simulink model "PID_quadricottero_v3"  (R2023b)
settings: Solver=VariableStepAuto  StartTime=0.0  StopTime=30  RelTol=1e-3
values from neighbouring files (symbols this model uses):
  b = 1.3e-5    (= 1.3e-05)    [data_quadricottero.m]
  d = 1.39e-6    (= 1.39e-06)    [data_quadricottero.m]
  g = 9.8    [data_quadricottero.m]
  Ix = 0.4    [data_quadricottero.m]
  Iy = 0.4    [data_quadricottero.m]
  Iz = 0.7    [data_quadricottero.m]
  l = 0.2    [data_quadricottero.m]
  m = 10    [data_quadricottero.m]
  p0 = 0    [data_quadricottero.m]
  phi0 = 0    [data_quadricottero.m]
  psi0 = 0    [data_quadricottero.m]
  q0 = 0    [data_quadricottero.m]
  r0 = 0    [data_quadricottero.m]
  Tc_Mx = 0.052    [data_quadricottero.m]
  theta0 = 0    [data_quadricottero.m]
libraries: simulink x2
settings Model: Creator=denin  LastModifiedBy=denin

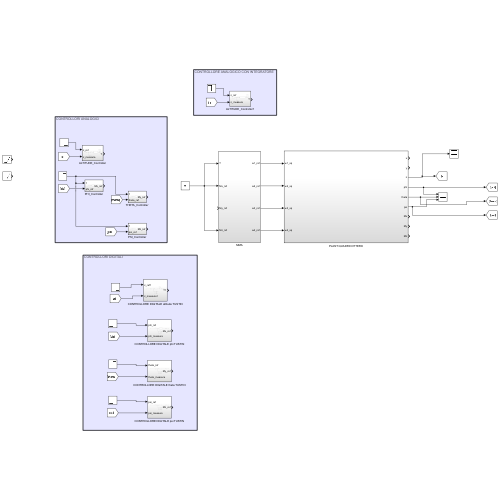
[thumbnail: Simulink's stored preview of the top-level diagram]
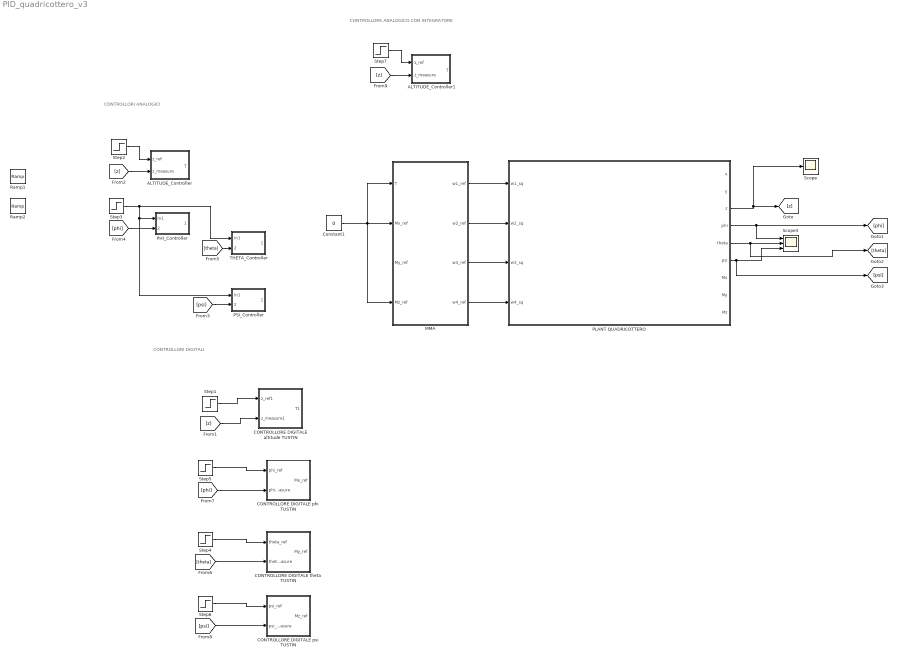
== system PID_quadricottero_v3 ==
  note: CONTROLLORE ANALOGICO CON INTEGRATORE
  note: CONTROLLORI ANALOGICI
  note: CONTROLLORI DIGITALI
  ALTITUDE_Controller : Subsystem
  ALTITUDE_Controller1 : Subsystem
  CONTROLLORE DIGITALE altitude TUSTIN : Subsystem
  CONTROLLORE DIGITALE phi TUSTIN : Subsystem
  CONTROLLORE DIGITALE psi TUSTIN : Subsystem
  CONTROLLORE DIGITALE theta TUSTIN : Subsystem
  Constant1 : Constant  Value=0
  MMA : Subsystem
  PHI_Controller : Subsystem
  PLANT QUADRICOTTERO : Subsystem
  PSI_Controller : Subsystem
  Ramp1 : simulink/Sources/Ramp  slope=1  start=0  InitialOutput=0
  Ramp2 : simulink/Sources/Ramp  slope=1  start=0  InitialOutput=0
  Scope : Scope
  Scope3 : Scope  NumInputPorts=3
  Step1 : Step  Time=0  After=-1  SampleTime=0
  Step2 : Step  Time=0  After=-1  SampleTime=0
  Step3 : Step  Time=0  SampleTime=0
  Step4 : Step  Time=0  After=10  SampleTime=0
  Step5 : Step  Time=0  SampleTime=0
  Step6 : Step  Time=0  SampleTime=0
  Step7 : Step  Time=0  After=-1  SampleTime=0
  THETA_Controller : Subsystem
  wires:
  PLANT QUADRICOTTERO/3(z) -> [z], Scope/1
  MMA/3(w3_ref) -> PLANT QUADRICOTTERO/3(w3_sq)
  MMA/4(w4_ref) -> PLANT QUADRICOTTERO/4(w4_sq)
  MMA/2(w2_ref) -> PLANT QUADRICOTTERO/2(w2_sq)
  MMA/1(w1_ref) -> PLANT QUADRICOTTERO/1(w1_sq)
  PLANT QUADRICOTTERO/4(phi) -> [phi], Scope3/1
  PLANT QUADRICOTTERO/5(theta) -> [theta], Scope3/2
  PLANT QUADRICOTTERO/6(psi) -> [psi], Scope3/3
  Step2/1 -> ALTITUDE_Controller/1(z_ref)
  [z] -> ALTITUDE_Controller/2(z_measure)
  Step3/1 -> PSI_Controller/1(In1), PHI_Controller/1(In1), THETA_Controller/1(In1)
  [phi] -> PHI_Controller/2(phi_ref)
  Constant1/1 -> MMA/2(Mx_ref), MMA/4(Mz_ref), MMA/1(T)
  [theta] -> THETA_Controller/2(theta_ref)
  [psi] -> PSI_Controller/2(psi_ref)
  Step1/1 -> CONTROLLORE DIGITALE altitude TUSTIN/1(z_ref1)
  [z] -> CONTROLLORE DIGITALE altitude TUSTIN/2(z_measure1)
  [phi] -> CONTROLLORE DIGITALE phi TUSTIN/2(phi_measure)
  Step5/1 -> CONTROLLORE DIGITALE phi TUSTIN/1(phi_ref)
  Step4/1 -> CONTROLLORE DIGITALE theta TUSTIN/1(theta_ref)
  [theta] -> CONTROLLORE DIGITALE theta TUSTIN/2(theta_measure)
  [psi] -> CONTROLLORE DIGITALE psi TUSTIN/2(psi_measure)
  Step6/1 -> CONTROLLORE DIGITALE psi TUSTIN/1(psi_ref)
  Step7/1 -> ALTITUDE_Controller1/1(z_ref)
  [z] -> ALTITUDE_Controller1/2(z_measure)

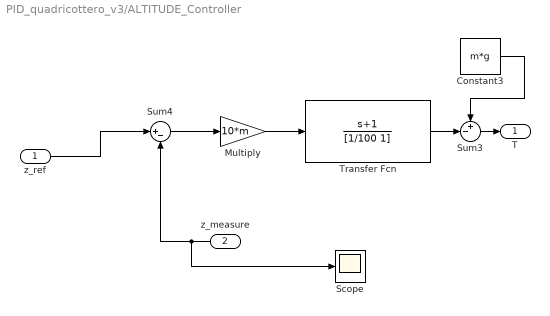
== system PID_quadricottero_v3/ALTITUDE_Controller ==
  z_ref : Inport
  z_measure : Inport  Port=2
  Constant3 : Constant  Value=m*g
  Multiply : Gain  Gain=10*m
  Scope : Scope
  Sum3 : Sum  Inputs=+-|
  Sum4 : Sum  Inputs=|+-
  Transfer Fcn : TransferFcn  Numerator=[1 1]  Denominator=[1/100 1]
  T : Outport
  wires:
  Multiply/1 -> Transfer Fcn/1
  Constant3/1 -> Sum3/1
  Sum4/1 -> Multiply/1
  z_measure/1 -> Scope/1, Sum4/2
  Sum3/1 -> T/1
  Transfer Fcn/1 -> Sum3/2
  z_ref/1 -> Sum4/1

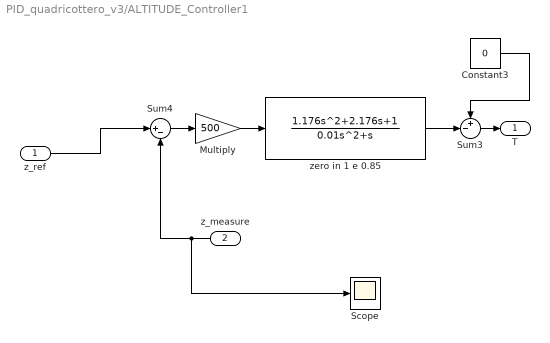
== system PID_quadricottero_v3/ALTITUDE_Controller1 ==
  z_ref : Inport
  z_measure : Inport  Port=2
  Constant3 : Constant  Value=0
  Multiply : Gain  Gain=500
  Scope : Scope
  Sum3 : Sum  Inputs=+-|
  Sum4 : Sum  Inputs=|+-
  zero in 1 e 0.85 : TransferFcn  Numerator=[1.176 2.176 1]  Denominator=[0.01 1 0]
  T : Outport
  wires:
  Constant3/1 -> Sum3/1
  Sum4/1 -> Multiply/1
  z_measure/1 -> Scope/1, Sum4/2
  Sum3/1 -> T/1
  z_ref/1 -> Sum4/1
  Multiply/1 -> zero in 1 e 0.85/1
  zero in 1 e 0.85/1 -> Sum3/2

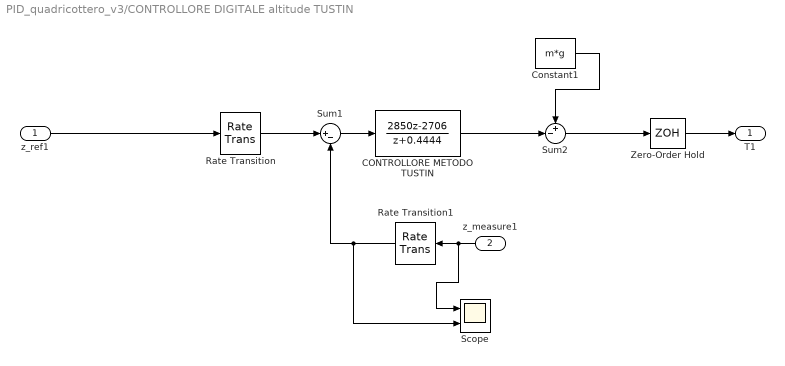
== system PID_quadricottero_v3/CONTROLLORE DIGITALE altitude TUSTIN ==
  z_ref1 : Inport
  z_measure1 : Inport  Port=2
  CONTROLLORE METODO TUSTIN : DiscreteTransferFcn  Numerator=[2850 -2706]  Denominator=[1 0.4444]
  Constant1 : Constant  Value=m*g
  Rate Transition : RateTransition  OutPortSampleTime=0.052
  Rate Transition1 : RateTransition  OutPortSampleTime=0.052
  Scope : Scope  NumInputPorts=2
  Sum1 : Sum  Inputs=|+-
  Sum2 : Sum  Inputs=+-|
  Zero-Order Hold : ZeroOrderHold  SampleTime=0.052
  T1 : Outport
  wires:
  z_ref1/1 -> Rate Transition/1
  z_measure1/1 -> Scope/1, Rate Transition1/1
  Rate Transition/1 -> Sum1/1
  Rate Transition1/1 -> Scope/2, Sum1/2
  Sum1/1 -> CONTROLLORE METODO TUSTIN/1
  Constant1/1 -> Sum2/1
  CONTROLLORE METODO TUSTIN/1 -> Sum2/2
  Sum2/1 -> Zero-Order Hold/1
  Zero-Order Hold/1 -> T1/1

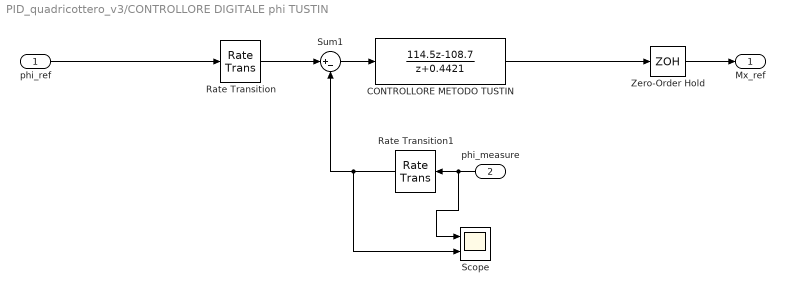
== system PID_quadricottero_v3/CONTROLLORE DIGITALE phi TUSTIN ==
  phi_ref : Inport
  phi_measure : Inport  Port=2
  CONTROLLORE METODO TUSTIN : DiscreteTransferFcn  Numerator=[114.5 -108.7]  Denominator=[1 0.4421]
  Rate Transition : RateTransition  OutPortSampleTime=Tc_Mx
  Rate Transition1 : RateTransition  OutPortSampleTime=Tc_Mx
  Scope : Scope  NumInputPorts=2
  Sum1 : Sum  Inputs=|+-
  Zero-Order Hold : ZeroOrderHold  SampleTime=Tc_Mx
  Mx_ref : Outport
  wires:
  phi_ref/1 -> Rate Transition/1
  phi_measure/1 -> Scope/1, Rate Transition1/1
  Rate Transition/1 -> Sum1/1
  Rate Transition1/1 -> Scope/2, Sum1/2
  Sum1/1 -> CONTROLLORE METODO TUSTIN/1
  CONTROLLORE METODO TUSTIN/1 -> Zero-Order Hold/1
  Zero-Order Hold/1 -> Mx_ref/1

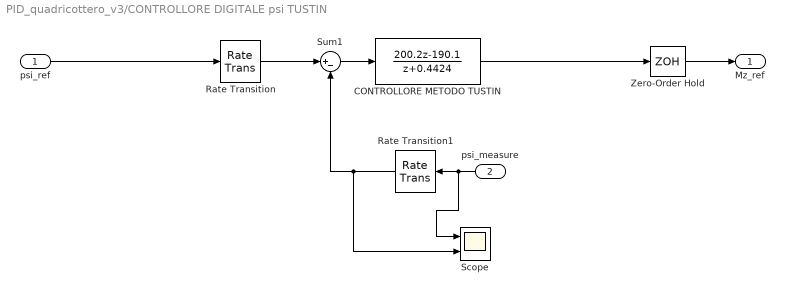
== system PID_quadricottero_v3/CONTROLLORE DIGITALE psi TUSTIN ==
  psi_ref : Inport
  psi_measure : Inport  Port=2
  CONTROLLORE METODO TUSTIN : DiscreteTransferFcn  Numerator=[200.2 -190.1]  Denominator=[1 0.4424]
  Rate Transition : RateTransition  OutPortSampleTime=Tc_Mx
  Rate Transition1 : RateTransition  OutPortSampleTime=Tc_Mx
  Scope : Scope  NumInputPorts=2
  Sum1 : Sum  Inputs=|+-
  Zero-Order Hold : ZeroOrderHold  SampleTime=Tc_Mx
  Mz_ref : Outport
  wires:
  psi_ref/1 -> Rate Transition/1
  psi_measure/1 -> Scope/1, Rate Transition1/1
  Rate Transition/1 -> Sum1/1
  Rate Transition1/1 -> Scope/2, Sum1/2
  Sum1/1 -> CONTROLLORE METODO TUSTIN/1
  CONTROLLORE METODO TUSTIN/1 -> Zero-Order Hold/1
  Zero-Order Hold/1 -> Mz_ref/1

== system PID_quadricottero_v3/CONTROLLORE DIGITALE theta TUSTIN ==
  theta_ref : Inport
  theta_measure : Inport  Port=2
  CONTROLLORE METODO TUSTIN : DiscreteTransferFcn  Numerator=[114.5 -108.7]  Denominator=[1 0.4421]
  Rate Transition : RateTransition  OutPortSampleTime=Tc_Mx
  Rate Transition1 : RateTransition  OutPortSampleTime=Tc_Mx
  Scope : Scope  NumInputPorts=2
  Sum1 : Sum  Inputs=|+-
  Zero-Order Hold : ZeroOrderHold  SampleTime=Tc_Mx
  My_ref : Outport
  wires:
  theta_ref/1 -> Rate Transition/1
  theta_measure/1 -> Scope/1, Rate Transition1/1
  Rate Transition/1 -> Sum1/1
  Rate Transition1/1 -> Scope/2, Sum1/2
  Sum1/1 -> CONTROLLORE METODO TUSTIN/1
  CONTROLLORE METODO TUSTIN/1 -> Zero-Order Hold/1
  Zero-Order Hold/1 -> My_ref/1

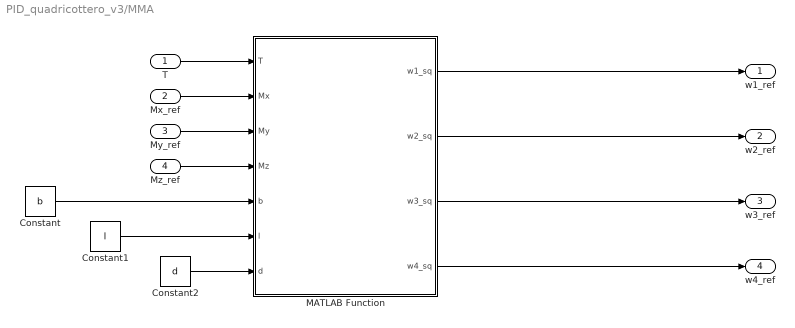
== system PID_quadricottero_v3/MMA ==
  T : Inport
  Mx_ref : Inport  Port=2
  My_ref : Inport  Port=3
  Mz_ref : Inport  Port=4
  Constant : Constant  Value=b
  Constant1 : Constant  Value=l
  Constant2 : Constant  Value=d
  MATLAB Function : MATLAB Function  TreatAsAtomicUnit=on
  w1_ref : Outport
  w2_ref : Outport  Port=2
  w3_ref : Outport  Port=3
  w4_ref : Outport  Port=4
  wires:
  Mz_ref/1 -> MATLAB Function/4(Mz)
  Constant2/1 -> MATLAB Function/7(d)
  Constant1/1 -> MATLAB Function/6(l)
  Constant/1 -> MATLAB Function/5(b)
  MATLAB Function/1(w1_sq) -> w1_ref/1
  MATLAB Function/2(w2_sq) -> w2_ref/1
  MATLAB Function/3(w3_sq) -> w3_ref/1
  MATLAB Function/4(w4_sq) -> w4_ref/1
  My_ref/1 -> MATLAB Function/3(My)
  Mx_ref/1 -> MATLAB Function/2(Mx)
  T/1 -> MATLAB Function/1(T)

== system PID_quadricottero_v3/PHI_Controller ==
  In1 : Inport
  phi_ref : Inport  Port=2
  Multiply1 : Gain  Gain=10*Ix
  Sum6 : Sum  Inputs=|+-
  Transfer Fcn1 : TransferFcn  Numerator=[1 1]  Denominator=[1/100 1]
  Mx_ref : Outport
  wires:
  Sum6/1 -> Multiply1/1
  Multiply1/1 -> Transfer Fcn1/1
  In1/1 -> Sum6/1
  phi_ref/1 -> Sum6/2
  Transfer Fcn1/1 -> Mx_ref/1

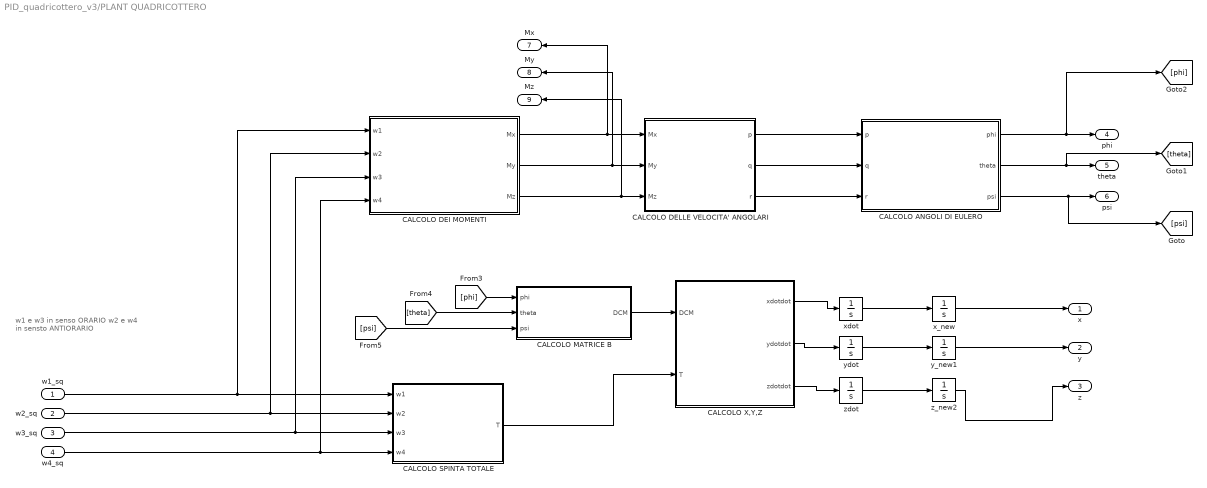
== system PID_quadricottero_v3/PLANT QUADRICOTTERO ==
  note: w1 e w3 in senso ORARIO
      | w2 e w4 in sensto ANTIORARIO
  w1_sq : Inport
  w2_sq : Inport  Port=2
  w3_sq : Inport  Port=3
  w4_sq : Inport  Port=4
  CALCOLO ANGOLI DI EULERO : Subsystem
  CALCOLO DEI MOMENTI : Subsystem
  CALCOLO DELLE VELOCITA' ANGOLARI : Subsystem
  CALCOLO MATRICE B : Subsystem
  CALCOLO SPINTA TOTALE : Subsystem
  CALCOLO X,Y,Z : Subsystem
  x_new : Integrator
  xdot : Integrator
  y_new1 : Integrator
  ydot : Integrator
  z_new2 : Integrator  UpperSaturationLimit=98  LowerSaturationLimit=-98
  zdot : Integrator  UpperSaturationLimit=98  LowerSaturationLimit=-98
  x : Outport
  y : Outport  Port=2
  z : Outport  Port=3
  phi : Outport  Port=4
  theta : Outport  Port=5
  psi : Outport  Port=6
  Mx : Outport  Port=7
  My : Outport  Port=8
  Mz : Outport  Port=9
  wires:
  CALCOLO DELLE VELOCITA' ANGOLARI/1(p) -> CALCOLO ANGOLI DI EULERO/1(p)
  CALCOLO X,Y,Z/1(xdotdot) -> xdot/1
  CALCOLO SPINTA TOTALE/1(T) -> CALCOLO X,Y,Z/2(T)
  CALCOLO X,Y,Z/3(zdotdot) -> zdot/1
  CALCOLO ANGOLI DI EULERO/3(psi) -> [psi], psi/1
  CALCOLO ANGOLI DI EULERO/2(theta) -> [theta], theta/1
  CALCOLO X,Y,Z/2(ydotdot) -> ydot/1
  CALCOLO DELLE VELOCITA' ANGOLARI/3(r) -> CALCOLO ANGOLI DI EULERO/3(r)
  CALCOLO DELLE VELOCITA' ANGOLARI/2(q) -> CALCOLO ANGOLI DI EULERO/2(q)
  CALCOLO MATRICE B/1(DCM) -> CALCOLO X,Y,Z/1(DCM)
  CALCOLO DEI MOMENTI/1(Mx) -> Mx/1, CALCOLO DELLE VELOCITA' ANGOLARI/1(Mx)
  CALCOLO DEI MOMENTI/2(My) -> My/1, CALCOLO DELLE VELOCITA' ANGOLARI/2(My)
  CALCOLO DEI MOMENTI/3(Mz) -> Mz/1, CALCOLO DELLE VELOCITA' ANGOLARI/3(Mz)
  w4_sq/1 -> CALCOLO DEI MOMENTI/4(w4), CALCOLO SPINTA TOTALE/4(w4)
  w3_sq/1 -> CALCOLO DEI MOMENTI/3(w3), CALCOLO SPINTA TOTALE/3(w3)
  w2_sq/1 -> CALCOLO DEI MOMENTI/2(w2), CALCOLO SPINTA TOTALE/2(w2)
  w1_sq/1 -> CALCOLO DEI MOMENTI/1(w1), CALCOLO SPINTA TOTALE/1(w1)
  CALCOLO ANGOLI DI EULERO/1(phi) -> [phi], phi/1
  xdot/1 -> x_new/1
  x_new/1 -> x/1
  ydot/1 -> y_new1/1
  y_new1/1 -> y/1
  zdot/1 -> z_new2/1
  [phi] -> CALCOLO MATRICE B/1(phi)
  [theta] -> CALCOLO MATRICE B/2(theta)
  [psi] -> CALCOLO MATRICE B/3(psi)
  z_new2/1 -> z/1

== system PID_quadricottero_v3/PSI_Controller ==
  In1 : Inport
  psi_ref : Inport  Port=2
  Multiply1 : Gain  Gain=10*Iz
  Sum6 : Sum  Inputs=|+-
  Transfer Fcn1 : TransferFcn  Numerator=[1 1]  Denominator=[1/100 1]
  Mz_ref : Outport
  wires:
  Sum6/1 -> Multiply1/1
  Multiply1/1 -> Transfer Fcn1/1
  In1/1 -> Sum6/1
  psi_ref/1 -> Sum6/2
  Transfer Fcn1/1 -> Mz_ref/1

== system PID_quadricottero_v3/THETA_Controller ==
  In1 : Inport
  theta_ref : Inport  Port=2
  Multiply1 : Gain  Gain=10*Iy
  Sum6 : Sum  Inputs=|+-
  Transfer Fcn1 : TransferFcn  Numerator=[1 1]  Denominator=[1/100 1]
  My_ref : Outport
  wires:
  Sum6/1 -> Multiply1/1
  Multiply1/1 -> Transfer Fcn1/1
  In1/1 -> Sum6/1
  theta_ref/1 -> Sum6/2
  Transfer Fcn1/1 -> My_ref/1

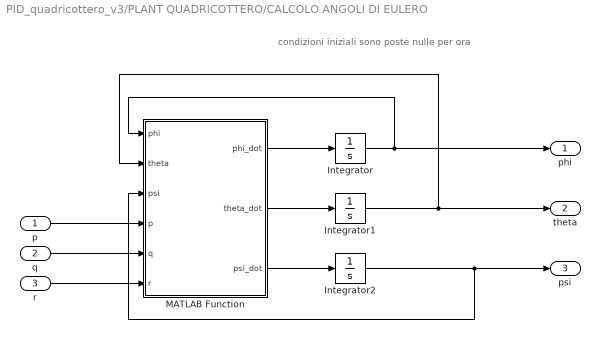
== system PID_quadricottero_v3/PLANT QUADRICOTTERO/CALCOLO ANGOLI DI EULERO ==
  note: condizioni iniziali sono poste nulle per ora
  p : Inport
  q : Inport  Port=2
  r : Inport  Port=3
  Integrator : Integrator  InitialCondition=phi0
  Integrator1 : Integrator  InitialCondition=theta0
  Integrator2 : Integrator  InitialCondition=psi0
  MATLAB Function : MATLAB Function  TreatAsAtomicUnit=on
  phi : Outport
  theta : Outport  Port=2
  psi : Outport  Port=3
  wires:
  Integrator2/1 -> MATLAB Function/3(psi), psi/1
  Integrator1/1 -> MATLAB Function/2(theta), theta/1
  Integrator/1 -> MATLAB Function/1(phi), phi/1
  p/1 -> MATLAB Function/4(p)
  q/1 -> MATLAB Function/5(q)
  r/1 -> MATLAB Function/6(r)
  MATLAB Function/1(phi_dot) -> Integrator/1
  MATLAB Function/3(psi_dot) -> Integrator2/1
  MATLAB Function/2(theta_dot) -> Integrator1/1

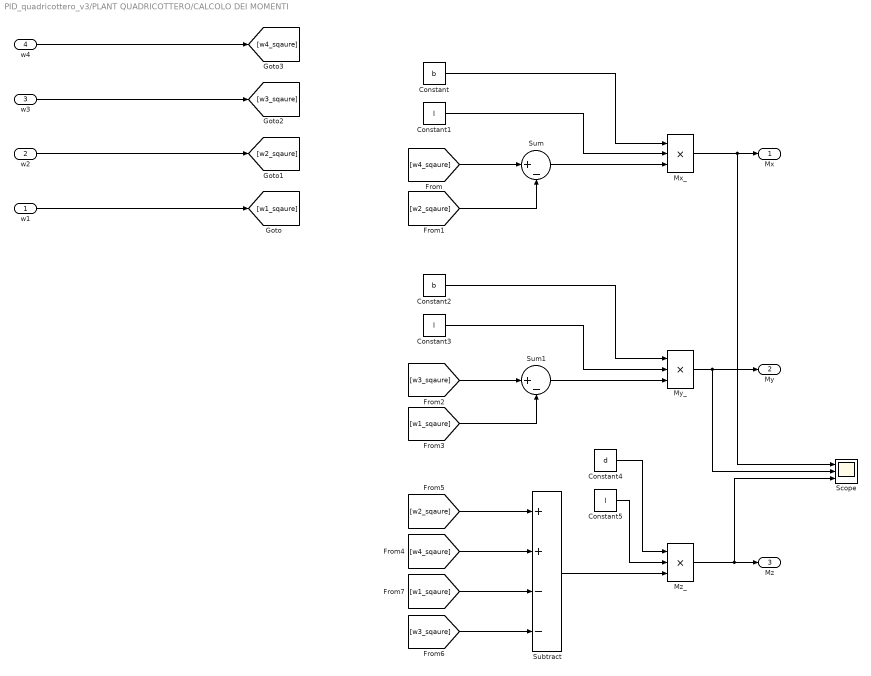
== system PID_quadricottero_v3/PLANT QUADRICOTTERO/CALCOLO DEI MOMENTI ==
  w1 : Inport
  w2 : Inport  Port=2
  w3 : Inport  Port=3
  w4 : Inport  Port=4
  Constant : Constant  Value=b
  Constant1 : Constant  Value=l
  Constant2 : Constant  Value=b
  Constant3 : Constant  Value=l
  Constant4 : Constant  Value=d
  Constant5 : Constant  Value=l
  Mx_ : Product  Inputs=3
  My_ : Product  Inputs=3
  Mz_ : Product  Inputs=3
  Scope : Scope  NumInputPorts=3
  Subtract : Sum  Inputs=++--
  Sum : Sum  Inputs=|+-
  Sum1 : Sum  Inputs=|+-
  Mx : Outport
  My : Outport  Port=2
  Mz : Outport  Port=3
  wires:
  w1/1 -> [w1_sqaure]
  w2/1 -> [w2_sqaure]
  w3/1 -> [w3_sqaure]
  w4/1 -> [w4_sqaure]
  [w2_sqaure] -> Sum/2
  [w4_sqaure] -> Sum/1
  Constant/1 -> Mx_/1
  Constant1/1 -> Mx_/2
  Sum/1 -> Mx_/3
  Mx_/1 -> Scope/1, Mx/1
  Constant2/1 -> My_/1
  Sum1/1 -> My_/3
  Constant3/1 -> My_/2
  My_/1 -> Scope/2, My/1
  [w2_sqaure] -> Subtract/1
  [w4_sqaure] -> Subtract/2
  [w1_sqaure] -> Subtract/3
  [w3_sqaure] -> Subtract/4
  Subtract/1 -> Mz_/3
  Constant4/1 -> Mz_/1
  Constant5/1 -> Mz_/2
  Mz_/1 -> Scope/3, Mz/1
  [w1_sqaure] -> Sum1/2
  [w3_sqaure] -> Sum1/1

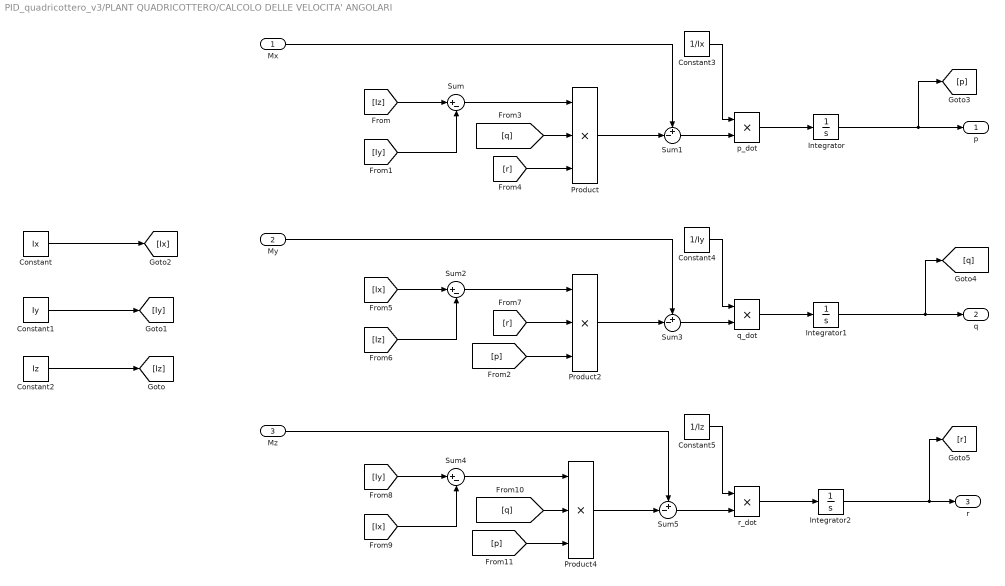
== system PID_quadricottero_v3/PLANT QUADRICOTTERO/CALCOLO DELLE VELOCITA' ANGOLARI ==
  Mx : Inport
  My : Inport  Port=2
  Mz : Inport  Port=3
  Constant : Constant  Value=Ix
  Constant1 : Constant  Value=Iy
  Constant2 : Constant  Value=Iz
  Constant3 : Constant  Value=1/Ix
  Constant4 : Constant  Value=1/Iy
  Constant5 : Constant  Value=1/Iz
  Integrator : Integrator  InitialCondition=p0
  Integrator1 : Integrator  InitialCondition=q0
  Integrator2 : Integrator  InitialCondition=r0
  Product : Product  Inputs=3
  Product2 : Product  Inputs=3
  Product4 : Product  Inputs=3
  Sum : Sum  Inputs=|+-
  Sum1 : Sum  Inputs=+-|
  Sum2 : Sum  Inputs=|+-
  Sum3 : Sum  Inputs=+-|
  Sum4 : Sum  Inputs=|+-
  Sum5 : Sum  Inputs=+-|
  p_dot : Product
  q_dot : Product
  r_dot : Product
  p : Outport
  q : Outport  Port=2
  r : Outport  Port=3
  wires:
  Constant1/1 -> [Iy]
  Constant2/1 -> [Iz]
  Constant/1 -> [Ix]
  [Iy] -> Sum/2
  [Iz] -> Sum/1
  Sum/1 -> Product/1
  Product/1 -> Sum1/2
  Mx/1 -> Sum1/1
  Sum1/1 -> p_dot/2
  Constant3/1 -> p_dot/1
  p_dot/1 -> Integrator/1
  Integrator/1 -> [p], p/1
  Integrator2/1 -> r/1, [r]
  [q] -> Product/2
  [r] -> Product/3
  [Iz] -> Sum2/2
  Sum2/1 -> Product2/1
  [Ix] -> Sum2/1
  Product2/1 -> Sum3/2
  Sum3/1 -> q_dot/2
  [r] -> Product2/2
  [p] -> Product2/3
  My/1 -> Sum3/1
  Constant4/1 -> q_dot/1
  q_dot/1 -> Integrator1/1
  Integrator1/1 -> [q], q/1
  Sum4/1 -> Product4/1
  [Iy] -> Sum4/1
  [Ix] -> Sum4/2
  [p] -> Product4/3
  [q] -> Product4/2
  Mz/1 -> Sum5/1
  Product4/1 -> Sum5/2
  Constant5/1 -> r_dot/1
  r_dot/1 -> Integrator2/1
  Sum5/1 -> r_dot/2

== system PID_quadricottero_v3/PLANT QUADRICOTTERO/CALCOLO MATRICE B ==
  phi : Inport
  theta : Inport  Port=2
  psi : Inport  Port=3
  MATLAB Function : MATLAB Function  TreatAsAtomicUnit=on
  DCM : Outport
  wires:
  MATLAB Function/1(DCM) -> DCM/1
  phi/1 -> MATLAB Function/1(phi)
  theta/1 -> MATLAB Function/2(theta)
  psi/1 -> MATLAB Function/3(psi)

== system PID_quadricottero_v3/PLANT QUADRICOTTERO/CALCOLO SPINTA TOTALE ==
  w1 : Inport
  w2 : Inport  Port=2
  w3 : Inport  Port=3
  w4 : Inport  Port=4
  Constant : Constant  Value=b
  Product : Product
  Subtract3 : Sum  Inputs=++++
  T : Outport
  wires:
  w4/1 -> Subtract3/4
  w2/1 -> Subtract3/2
  w1/1 -> Subtract3/1
  w3/1 -> Subtract3/3
  Subtract3/1 -> Product/2
  Constant/1 -> Product/1
  Product/1 -> T/1

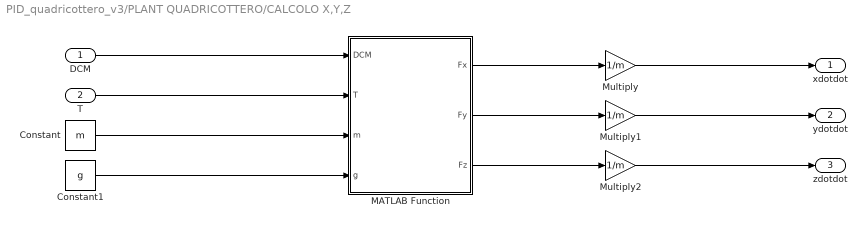
== system PID_quadricottero_v3/PLANT QUADRICOTTERO/CALCOLO X,Y,Z ==
  DCM : Inport
  T : Inport  Port=2
  Constant : Constant  Value=m
  Constant1 : Constant  Value=g
  MATLAB Function : MATLAB Function  TreatAsAtomicUnit=on
  Multiply : Gain  Gain=1/m
  Multiply1 : Gain  Gain=1/m
  Multiply2 : Gain  Gain=1/m
  xdotdot : Outport
  ydotdot : Outport  Port=2
  zdotdot : Outport  Port=3
  wires:
  MATLAB Function/3(Fz) -> Multiply2/1
  MATLAB Function/2(Fy) -> Multiply1/1
  MATLAB Function/1(Fx) -> Multiply/1
  DCM/1 -> MATLAB Function/1(DCM)
  T/1 -> MATLAB Function/2(T)
  Constant/1 -> MATLAB Function/3(m)
  Constant1/1 -> MATLAB Function/4(g)
  Multiply/1 -> xdotdot/1
  Multiply1/1 -> ydotdot/1
  Multiply2/1 -> zdotdot/1

== matlab function PID_quadricottero_v3/PLANT QUADRICOTTERO/CALCOLO ANGOLI DI EULERO/MATLAB Function ==
  data: phi input; phi_dot output; theta input; psi input; p input; q input; r input; theta_dot output; psi_dot output
function [phi_dot, theta_dot, psi_dot] = fcn(phi,theta,psi,p,q,r)


ROT =  [1   sin(phi)*tan(theta)  cos(phi)*tan(theta);
        0   cos(phi)            -sin(phi);
        0   sin(phi)/cos(theta) cos(phi)/cos(theta);];

dot = ROT*[p; q; r];

phi_dot = dot(1,1);
theta_dot = dot(2,1);
psi_dot = dot(3,1);

== matlab function PID_quadricottero_v3/PLANT QUADRICOTTERO/CALCOLO MATRICE B/MATLAB Function ==
  data: phi input; DCM output; theta input; psi input
function DCM  = fcn(phi, theta, psi)

DCM =  [cos(theta)*cos(psi)     -cos(phi)*sin(psi)+sin(phi)*sin(theta)*cos(psi)      sin(phi)*sin(psi)+cos(phi)*sin(theta)*cos(psi);
        cos(theta)*sin(psi)    cos(phi)*cos(psi)+sin(phi)*sin(theta)*sin(psi)      -sin(phi)*cos(psi)+cos(phi)*sin(theta)*sin(psi);
        -sin(theta)              sin(phi)*cos(theta)                                cos(phi)*cos(theta)];

== matlab function PID_quadricottero_v3/PLANT QUADRICOTTERO/CALCOLO X,Y,Z/MATLAB Function ==
  data: DCM input; Fx output; T input; m input; g input; Fy output; Fz output
function [Fx, Fy, Fz] = fcn(DCM, T, m, g)

F = [0; 0; m*g] - DCM*[0; 0; T];

Fx = F(1,1);
Fy = F(2,1);
Fz = F(3,1);

== matlab function PID_quadricottero_v3/MMA/MATLAB Function ==
  data: T input; w1_sq output; Mx input; My input; Mz input; w2_sq output; w3_sq output; w4_sq output; b input; l input; d input
function [w1_sq, w2_sq, w3_sq, w4_sq] = fcn(T, Mx, My, Mz, b, l, d)

matrix = [b     b       b       b;
         0      -l*b    0       l*b;
        -l*b    0       l*b     0;
        -l*d    l*d     -l*d    l*d];

motor_matrix = inv(matrix);
w_sq_matrix = motor_matrix*[T; Mx; My; Mz];

w1_sq = w_sq_matrix(1,1)
w2_sq = w_sq_matrix(2,1)
w3_sq = w_sq_matrix(3,1)
w4_sq = w_sq_matrix(4,1)
